simulink library "Quadrotor_tools"  (Simulink 8.0)
settings: Solver=ode45  StartTime=0.0  StopTime=10.0  RelTol=1e-3
libraries: Quadrotor_tools x3
settings Model: Creator=edredone  LastModifiedBy=leoas_000

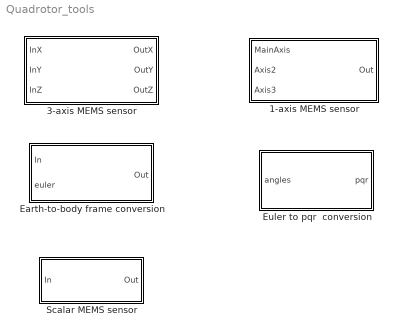
== system Quadrotor_tools ==
  1-axis MEMS sensor : Subsystem  mask(1-axis MEMS sensor){gain=0, gain2=0, gain3=0, b=0, var=0, seed=0, delay=0, isClipped=on, satUp=0, satLow=0}
      mask prompts: gain "Sensor gain:"; gain2 "Axis 2 interference gain:"; gain3 "Axis 3 interference gain;"; b "Sensor bias:"; var "Error variance:"; seed "Random seed for error generation:"; delay "Output delay:"; isClipped "Saturate output."; satUp "Saturation upper limit:"; satLow "Saturation lower limit:"
      mask help:
      | Simple model for a single axis MEMS sensor.
      | This sensor measures a vector quantity along one axis, but interferences
      | from the other axes are allowed to model misalignment related errors.
      | This sensor model does not take into account the voltage conversion,
      | the output value has the same dimensions of the input physical quantity.
      mask Display:
      | port_label('input', 1, 'MainAxis');
      | port_label('input', 2, 'Axis2');
      | port_label('input', 3, 'Axis3');
      | port_label('output', 1, 'Out');
  3-axis MEMS sensor : Subsystem  mask(3-axis MEMS sensor){biasX=0, biasY=0, biasZ=0, varX=0, varY=0, varZ=0, satUp=0, satLow=0, delay=0, sampleTime=0, gainX=[], gainY=0, gainZ=0, gainXY=0, gainXZ=0, gainYX=0, gainYZ=0, gainZX=0, gainZY=0, seedX=0, seedY=0, seedZ=0}
      mask prompts: biasX "x-axis bias:"; biasY "y-axis bias:"; biasZ "z-axis bias:"; varX "x-axis error variance:"; varY "y-axis error variance:"; varZ "z-axis error variance:"; satUp "Upper output saturation limit:"; satLow "Lower output saturation limit:"; delay "Output delay:"; sampleTime "Sample time (-1 for inherited):"; gainX "x-axis gain:"; gainY "y-axis gain:"; gainZ "z-axis gain:"; gainXY "X on Y misalignment factor:"; gainXZ "X on Z misalignment factor:"; gainYX "Y on X misalignment factor:"; gainYZ "Y on Z misalignment factor:"; gainZX "Z on X misalignment factor:"; gainZY "Z on Y misalignment factor:"; seedX "Random seed for x-axis error:"; seedY "Random seed for y-axis error:"; seedZ "Random seed for z-axis error:"
      mask help:
      | A simple model for a generic 3-axis MEMS sensor.
      | This sensor model does not take into account the voltage conversion,
      | the output value has the same dimensions of the input physical quantity.
      mask Display:
      | port_label('input', 1, 'InX');
      | port_label('input', 2, 'InY');
      | port_label('input', 3, 'InZ');
      | 
      | port_label('output', 1, 'OutX');
      | port_label('output', 2, 'OutY');
      | port_label('output', 3, 'OutZ');
  Earth-to-body frame conversion : Subsystem  mask(Earth-to-body frame conversion){}
      mask help:
      | Converts the components of a vector from the earth (fixed) frame to the
      | body frame, given the orientation of the body frame expressed with the
      | Euler angles.
      mask Display:
      | port_label('input', 1, 'v');
      | port_label('input', 2, '[phi theta psi]');
      | port_label('output', 1, 'v1');
  Euler to pqr  conversion : Subsystem  mask(Euler to pqr conversion){}
      mask help:
      | Computes the vector [p q r] of the angular velocity in the body frame
      | from the orientations espressed with the Euler angles.
      mask Display:
      | port_label('input', 1, '[phi theta psi]');
      | port_label('output', 1, 'pqr');
  Scalar MEMS sensor : Subsystem  mask{gain=0, bias=0, var=0, seed=0, isClipped=on, satUp=0, satLow=0, delay=0}
      mask prompts: var "Sensor noise variance:"; seed "Random seed for the sensor noise:"; isClipped "Saturate output:"; satUp "Upper saturation limit:"; satLow "Lower saturation limit:"; delay "Sensor response delay:"
      mask Display:
      | port_label('output', 1, 'out');
      | port_label('input', 1, 'in');

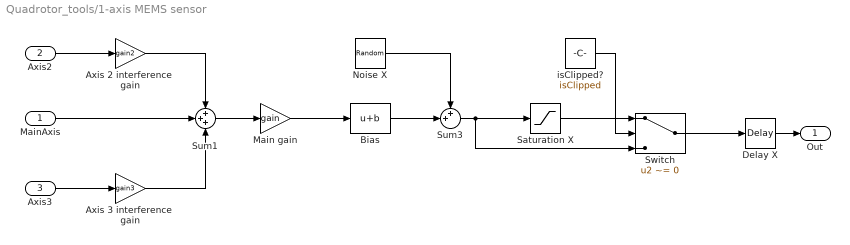
== system Quadrotor_tools/1-axis MEMS sensor ==
  MainAxis : Inport
  Axis2 : Inport  Port=2
  Axis3 : Inport  Port=3
  Axis 2 interference  gain : Gain  Gain=gain2
  Axis 3 interference  gain : Gain  Gain=gain3
  Bias : Bias  Bias=b
  Delay X : TransportDelay  DelayTime=delay
  Main gain : Gain  Gain=gain
  Noise X : RandomNumber  Variance=var  Seed=seed  SampleTime=0.001
  Saturation X : Saturate  UpperLimit=satUp  LowerLimit=satLow
  Sum1 : Sum  Inputs=+++
  Sum3 : Sum  Inputs=++|
  Switch : Switch  Criteria=u2 ~= 0
  isClipped? : Constant  Value=isClipped
  Out : Outport
  wires:
  Main gain/1 -> Bias/1
  Bias/1 -> Sum3/2
  Noise X/1 -> Sum3/1
  Sum3/1 -> Saturation X/1, Switch/3
  Delay X/1 -> Out/1
  Sum1/1 -> Main gain/1
  MainAxis/1 -> Sum1/2
  Axis 2 interference  gain/1 -> Sum1/1
  Axis 3 interference  gain/1 -> Sum1/3
  Axis2/1 -> Axis 2 interference  gain/1
  Axis3/1 -> Axis 3 interference  gain/1
  Saturation X/1 -> Switch/1
  Switch/1 -> Delay X/1
  isClipped?/1 -> Switch/2

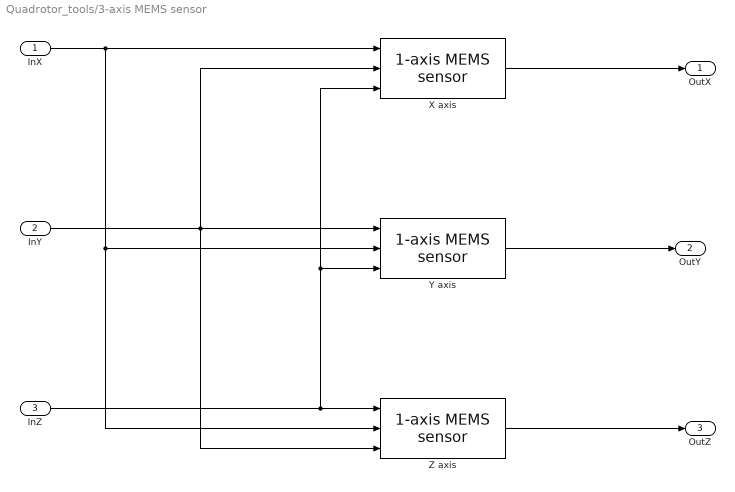
== system Quadrotor_tools/3-axis MEMS sensor ==
  InX : Inport
  InY : Inport  Port=2
  InZ : Inport  Port=3
  X axis : Quadrotor_tools/1-axis MEMS sensor  gain=gainX  gain2=gainXY  gain3=gainXZ  b=biasX  var=varX  seed=seedX  delay=delay  isClipped=on  satUp=satUp  satLow=satLow
  Y axis : Quadrotor_tools/1-axis MEMS sensor  gain=gainY  gain2=gainYX  gain3=gainYZ  b=biasY  var=varY  seed=seedY  delay=delay  isClipped=on  satUp=satUp  satLow=satLow
  Z axis : Quadrotor_tools/1-axis MEMS sensor  gain=gainZ  gain2=gainZX  gain3=gainZY  b=biasZ  var=varZ  seed=seedZ  delay=delay  isClipped=on  satUp=satUp  satLow=satLow
  OutX : Outport
  OutY : Outport  Port=2
  OutZ : Outport  Port=3
  wires:
  InX/1 -> X axis/1, Z axis/2, Y axis/2
  X axis/1 -> OutX/1
  InY/1 -> Y axis/1, X axis/2, Z axis/3
  Y axis/1 -> OutY/1
  InZ/1 -> Z axis/1, X axis/3, Y axis/3
  Z axis/1 -> OutZ/1

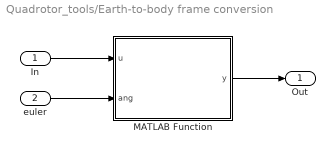
== system Quadrotor_tools/Earth-to-body frame conversion ==
  In : Inport
  euler : Inport  Port=2
  MATLAB Function : MATLAB Function  TreatAsAtomicUnit=on
  Out : Outport
  wires:
  In/1 -> MATLAB Function/1(u)
  MATLAB Function/1(y) -> Out/1
  euler/1 -> MATLAB Function/2(ang)

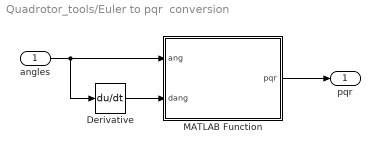
== system Quadrotor_tools/Euler to pqr  conversion ==
  angles : Inport
  Derivative : Derivative
  MATLAB Function : MATLAB Function  TreatAsAtomicUnit=on
  pqr : Outport
  wires:
  MATLAB Function/1(pqr) -> pqr/1
  angles/1 -> MATLAB Function/1(ang), Derivative/1
  Derivative/1 -> MATLAB Function/2(dang)

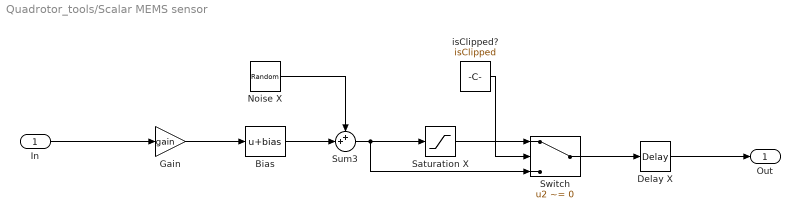
== system Quadrotor_tools/Scalar MEMS sensor ==
  In : Inport
  Bias : Bias  Bias=bias
  Delay X : TransportDelay  DelayTime=delay
  Gain : Gain  Gain=gain
  Noise X : RandomNumber  Variance=var  Seed=seed  SampleTime=0.001
  Saturation X : Saturate  UpperLimit=satUp  LowerLimit=satLow
  Sum3 : Sum  Inputs=++|
  Switch : Switch  Criteria=u2 ~= 0
  isClipped? : Constant  Value=isClipped
  Out : Outport
  wires:
  Gain/1 -> Bias/1
  Bias/1 -> Sum3/2
  Noise X/1 -> Sum3/1
  Sum3/1 -> Switch/3, Saturation X/1
  Delay X/1 -> Out/1
  Saturation X/1 -> Switch/1
  Switch/1 -> Delay X/1
  isClipped?/1 -> Switch/2
  In/1 -> Gain/1

== matlab function Earth-to-body frame conversion/MATLAB Function ==
  data u settings: description=Input vector
  data y settings: description=Output vector
  data ang settings: description=Euler angles.
  data: u input double size=3; y output double size=3; ang input double size=3
function y = fix2body(u, ang)
%#codegen
% ----------------------------------------------------
% This function converts the vector u from the earth
% frame to the body frame, given the orentation of the
% body in Euler angles.
% ----------------------------------------------------

% Euler angles
phi = ang(1);
theta = ang(2);
psi = ang(3);

% Rotation matrix
R = [cos(psi)*cos(theta), cos(psi)*sin(theta)*sin(phi)-sin(psi)*cos(phi),...
    cos(psi)*sin(theta)*cos(phi)+sin(psi)*sin(phi);
      sin(psi)*cos(theta), sin(psi)*sin(theta)*sin(phi)+cos(psi)*cos(phi),...
      sin(psi)*sin(theta)*cos(phi)-cos(psi)*sin(phi);
      -sin(theta) cos(theta)*sin(phi) cos(theta)*cos(phi)];

y = R'*u;

== matlab function Euler to pqr conversion/MATLAB Function ==
  data: ang input double; pqr output double; dang input double
function pqr = euler2pqr(ang, dang)
%#codegen
% ----------------------------------------------------
% This function converts the angular rates expressed
% in the earth frame to the body frame angular velocity
% components p, q and r. The function needs to know 
% also the orientation of the body frame in Euler 
% angles.
% ----------------------------------------------------

% Euler angles
phi = ang(1);
theta = ang(2);
% Note: the angle psi is not actually needed by the function.

A = [1 0 -sin(theta); 
     0 cos(phi) sin(phi)*cos(theta); 
     0 -sin(phi) cos(phi)*cos(theta)];

pqr = A*dang;
